simulink subsystem "AccelerationMaking"  (R2022b)
settings: Solver=VariableStepAuto  StartTime=0.0  StopTime=10.0  RelTol=1e-3
libraries: simulink x1
settings Model: Creator=hubkapatrik  LastModifiedBy=hubkapatrik

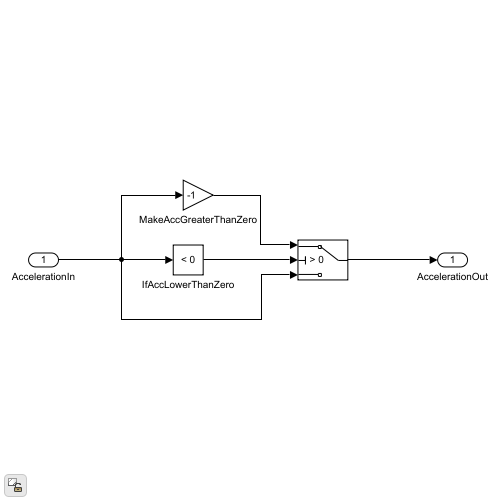
[thumbnail: Simulink's stored preview of the top-level diagram]
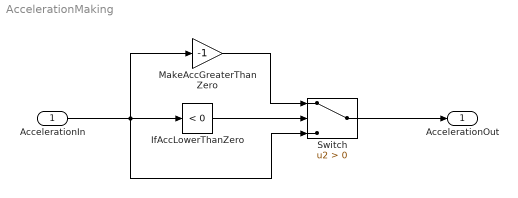
== system AccelerationMaking ==
  AccelerationIn : Inport
  IfAccLowerThanZero : simulink/Logic and Bit Operations/Compare To Constant  relop=<  const=0  OutDataTypeStr=boolean
  MakeAccGreaterThanZero : Gain  Gain=-1
  Switch : Switch  Criteria=u2 > Threshold  SaturateOnIntegerOverflow=off  InputSameDT=off
  AccelerationOut : Outport
  wires:
  AccelerationIn/1 -> MakeAccGreaterThanZero/1, Switch/3, IfAccLowerThanZero/1
  IfAccLowerThanZero/1 -> Switch/2
  MakeAccGreaterThanZero/1 -> Switch/1
  Switch/1 -> AccelerationOut/1
